simulink library "states_lib"  (R2022b)
settings: Solver=VariableStepAuto  StartTime=0.0  StopTime=10.0  RelTol=1e-3
undefined symbols (not defined in the file): raptor_xcp_function
libraries: Raptor_lib x3
settings Model: Creator=serga  LastModifiedBy=serga

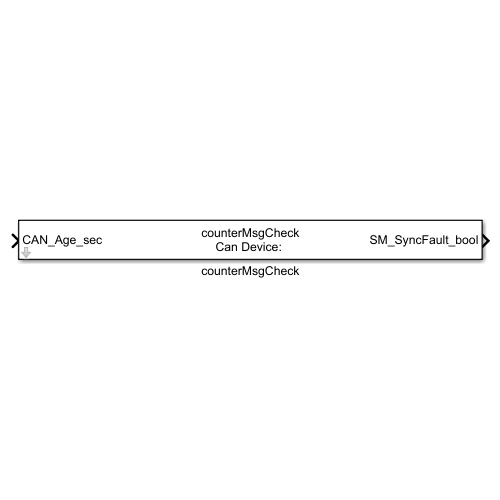
[thumbnail: Simulink's stored preview of the top-level diagram]
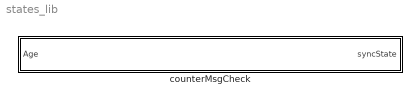
== system states_lib ==
  counterMsgCheck : Subsystem  mask{pos=''}
      mask prompts: pos "Can Node"
      mask Display:
      | disp(['counterMsgCheck\n' ...
      |     'Can Device: ' pos]);
      | port_label('input', 1, ['CAN_' pos 'Age_sec']);
      | port_label('output', 1, ['SM_' pos 'SyncFault_bool']);

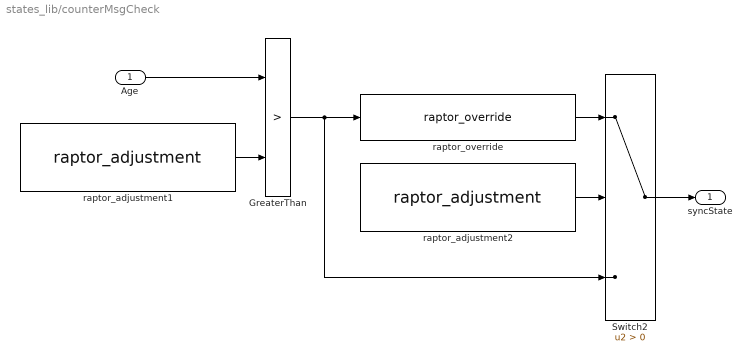
== system states_lib/counterMsgCheck ==
  Age : Inport
  GreaterThan : RelationalOperator  Operator=>  OutDataTypeStr=boolean  RndMeth=Simplest  InputSameDT=off
  Switch2 : Switch  Criteria=u2 > Threshold  SaturateOnIntegerOverflow=off  InputSameDT=off
  raptor_adjustment1 : Raptor_lib/Data Storage/raptor_adjustment  paramName=['SM_' pos 'CANFaultThresh_bool']  nameSource=Parameter  initValue=0  dataType=boolean  storage=Calibration  calDispType=Number  calEnum={'False', 'True'}  calGain=1.0  calOffset=0.0  calMax=inf  calMin=-inf  calFormat='-1'  calUnit=''  calHelp=''  calAccess=1  calFunction=raptor_xcp_function(gcb)  calDispHeaders=off  calColHeaders={'Col1' 'Col2' 'Col3'}  calRowHeaders={'Row1' 'Row2' 'Row3'}
      settings: SourceProductName=Raptor
  raptor_adjustment2 : Raptor_lib/Data Storage/raptor_adjustment  paramName=['SM_' pos 'CANFaultOverride_bool']  nameSource=Parameter  initValue=0  dataType=boolean  storage=Calibration  calDispType=Number  calEnum={'False', 'True'}  calGain=1.0  calOffset=0.0  calMax=inf  calMin=-inf  calFormat='-1'  calUnit=''  calHelp=''  calAccess=1  calFunction=raptor_xcp_function(gcb)  calDispHeaders=off  calColHeaders={'Col1' 'Col2' 'Col3'}  calRowHeaders={'Row1' 'Row2' 'Row3'}
      settings: SourceProductName=Raptor
  raptor_override : Raptor_lib/Data Storage/raptor_override  paramName=['SM_' pos 'CANFault_bool']  nameSource=Parameter  measurement=None  calDispType=Number  calEnum={'False', 'True'}  calGain=1.0  calOffset=0.0  calMax=inf  calMin=-inf  calFormat='-1'  calUnit=''  calHelp=''  calAccess=1  calFunction="[raptor_xcp_function(gcb) '|'  'Override']"
      settings: SourceProductName=Raptor
  syncState : Outport
  wires:
  GreaterThan/1 -> Switch2/3, raptor_override/1
  raptor_adjustment2/1 -> Switch2/2
  raptor_override/1 -> Switch2/1
  Switch2/1 -> syncState/1
  Age/1 -> GreaterThan/1
  raptor_adjustment1/1 -> GreaterThan/2
